simulink model "CAG_PH"  (R2020a)
settings: Solver=FixedStepAuto  StartTime=0.0  StopTime=10  FixedStep=1e-6  RelTol=1e-3  EnableMultiTasking=on
libraries: powerlib x23
settings Model: SimulationMode=accelerator  Creator=SINA  LastModifiedBy=ABO-CHIFA
settings DataIOCC: ReturnWorkspaceOutputs=off
settings OptimizationCC: LifeSpan=inf
settings DebuggingCC: SFUnexpectedBacktrackingDiag=warning  SFNoUnconditionalDefaultTransitionDiag=warning  ArithmeticOperatorsInVariantConditions=warning
settings SFSimCC: SimUseLocalCustomCode=off  CustomCodeUndefinedFunction=UseInterfaceOnly
settings RTWCC: RTWUseLocalCustomCode=off
settings CodeAppCC: StateflowObjectComments=on
settings GRTTargetCC: TargetLangStandard=C89/C90 (ANSI)
settings ConfigComp: CovMetricSettings=dw  CovHtmlReporting=on  CovSaveCumulativeToWorkspaceVar=on  CovSaveSingleToWorkspaceVar=on  CovExternalEMLEnable=off
settings SimscapeCC: SimscapeNormalizeSystem=off

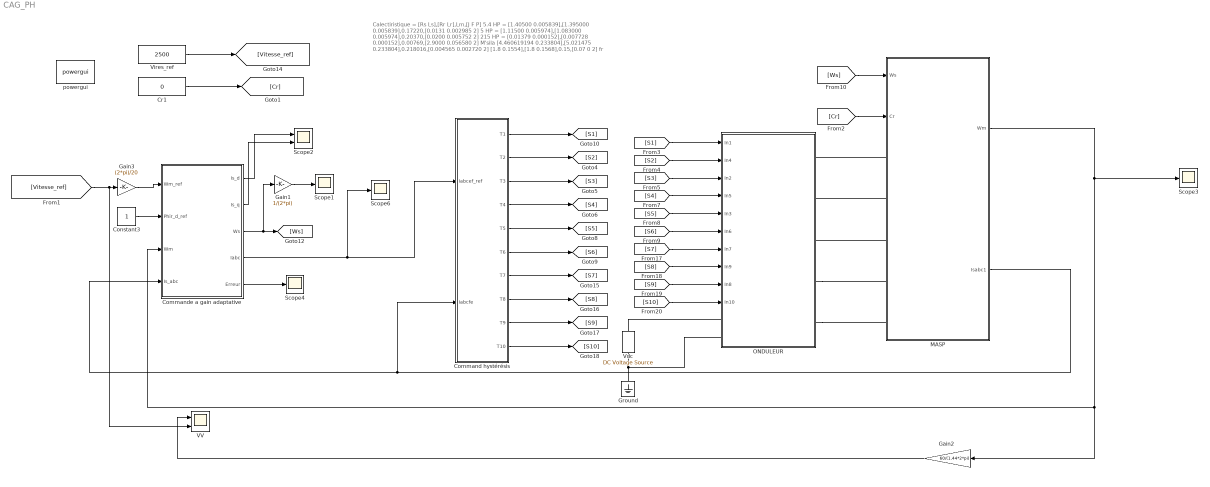
== system CAG_PH ==
  note: Calectiristique = [Rs Ls],[Rr Lr],Lm,[J F P]
      |
      | 5.4 HP = [1.40500 0.005839],[1.395000 0.005839],0.17220,[0.0131 0.002985 2]
      | 5 HP = [1.11500 0.005974],[1.083000 0.005974],0.20370,[0.0200 0.005752 2]
      | 215 HP = [0.01379 0.000152],[0.007728 0.000152],0.00769,[2.9000 0.056580 2]
      |
      | M'sila
      | [4.460619194 0.233804],[5.021475 0.233804],0.218016,[0.004565 0.002720 2]
      |
      | [1.8 0.1554],[1.8 0.1568],0.15,[0.07 0 2] fr
  Command hystérésis : Subsystem
  Commande a gain adaptative : Subsystem
  Constant3 : Constant
  Cr1 : Constant  Value=0
  Gain1 : Gain  Gain=1/(2*pi)
  Gain2 : Gain  Gain=60/(1.44*2*pi)
  Gain3 : Gain  Gain=(2*pi)/20
  Ground : powerlib/Elements/Ground  LConnTagsString=a
  MASP : Subsystem
  ONDULEUR : Subsystem
  Scope{1,3..4,6} (4 alike) : Scope
  Scope2 : Scope  NumInputPorts=2
  VV : Scope  NumInputPorts=2
  Vdc : powerlib/Electrical Sources/DC Voltage Source  Amplitude=650  Measurements=Voltage
  Vires_ref : Constant  Value=2500
  powergui : powerlib/powergui  Priority=1  SimulationMode=Discrete  SampleTime=1e-6  frequency=60  Iterations=50  frequencyindice=0  Pbase=100e6  ErrMax=1e-4  UnitsV=kV  UnitsW=MW  buscounter=0  FunctionMessages=off  echomessages=off  EnableUseOfTLC=off  CurrentSourceSwitches=off  DisableSnubberDevices=off  DisableRonSwitches=off  DisableVfSwitches=off  DisplayEquations=off  AutomaticDiscreteSolvers=off  SolverType=Tustin/Backward Euler (TBE)  Interpol=off  ExternalGateDelay=off  methode=off  Ts=0  x0status=blocks  SPID=off  SwTol=0  HookPort=off  NonlinearTolerance=1e-4  nMaxIteration=100  ContinueOnMaxIteration=off  RestoreLinks=warning  ResistiveCurrentMeasurement=off  Frange=[0:2:500]  Ylog=off  Xlog=on  ShowGrid=off  save=off  variable=ZData  structure=0  ZoomFFT=on  StartTime=0.0  cycles=1  DisplayStyle=1  fundamental=60  FreqAxis=off  MaxFrequency=1000  frequencyindicesteady=1  RmsSteady=1  display=off
  wires:
  Constant3/1 -> Commande a gain adaptative/2(Phir_d_ref)
  Commande a gain adaptative/3(Ws) -> [Ws], Gain1/1
  Commande a gain adaptative/4(Iabc) -> Command hystérésis/1(Iabcef_ref), Scope6/1
  Gain1/1 -> Scope1/1
  Commande a gain adaptative/1(Is_d) -> Scope2/1
  Commande a gain adaptative/2(Is_q) -> Scope2/2
  Commande a gain adaptative/5(Erreur) -> Scope4/1
  Cr1/1 -> [Cr]
  [Ws] -> MASP/1(Ws)
  [Cr] -> MASP/2(Cr)
  [Vitesse_ref] -> VV/2, Gain3/1
  Gain3/1 -> Commande a gain adaptative/1(Wm_ref)
  Gain2/1 -> VV/1
  MASP/1(Wm) -> Scope3/1, Gain2/1, Commande a gain adaptative/3(Wm)
  Vires_ref/1 -> [Vitesse_ref]
  [S1] -> ONDULEUR/1(In1)
  [S2] -> ONDULEUR/2(In4)
  [S10] -> ONDULEUR/10(In10)
  [S9] -> ONDULEUR/9(In8)
  [S3] -> ONDULEUR/3(In2)
  [S7] -> ONDULEUR/7(In7)
  [S6] -> ONDULEUR/6(In6)
  [S8] -> ONDULEUR/8(In9)
  [S4] -> ONDULEUR/4(In5)
  [S5] -> ONDULEUR/5(In3)
  Command hystérésis/2(T2) -> [S2]
  Command hystérésis/8(T8) -> [S8]
  Command hystérésis/9(T9) -> [S9]
  MASP/2(Isabc1) -> Command hystérésis/2(Iabcfe), Commande a gain adaptative/4(Is_abc)
  Command hystérésis/10(T10) -> [S10]
  Command hystérésis/1(T1) -> [S1]
  Command hystérésis/3(T3) -> [S3]
  Command hystérésis/5(T5) -> [S5]
  Command hystérésis/4(T4) -> [S4]
  Command hystérésis/7(T7) -> [S7]
  Command hystérésis/6(T6) -> [S6]
  connections:
  ONDULEUR/LConn2 -- Vdc/LConn1 -- Ground/LConn1
  Vdc/RConn1 -- ONDULEUR/LConn1
  MASP/LConn1 -- ONDULEUR/RConn1
  MASP/LConn2 -- ONDULEUR/RConn2
  MASP/LConn3 -- ONDULEUR/RConn3
  ONDULEUR/RConn4 -- MASP/LConn4
  ONDULEUR/RConn5 -- MASP/LConn5

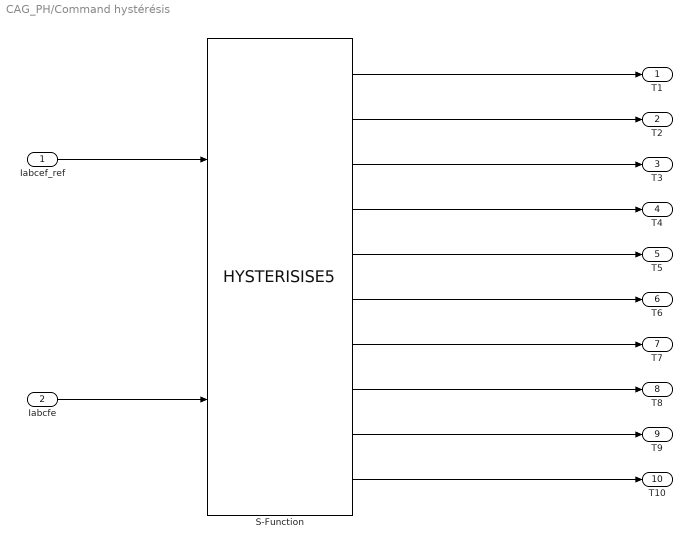
== system CAG_PH/Command hystérésis ==
  Iabcef_ref : Inport
  Iabcfe : Inport  Port=2
  S-Function : S-Function  FunctionName=HYSTERISISE5  Parameters=""  SFunctionDeploymentMode=off  EnableBusSupport=off
  T1 : Outport
  T2 : Outport  Port=2
  T3 : Outport  Port=3
  T4 : Outport  Port=4
  T5 : Outport  Port=5
  T6 : Outport  Port=6
  T7 : Outport  Port=7
  T8 : Outport  Port=8
  T9 : Outport  Port=9
  T10 : Outport  Port=10
  wires:
  Iabcef_ref/1 -> S-Function/1
  Iabcfe/1 -> S-Function/2
  S-Function/1 -> T1/1
  S-Function/2 -> T2/1
  S-Function/3 -> T3/1
  S-Function/4 -> T4/1
  S-Function/5 -> T5/1
  S-Function/6 -> T6/1
  S-Function/7 -> T7/1
  S-Function/8 -> T8/1
  S-Function/9 -> T9/1
  S-Function/10 -> T10/1

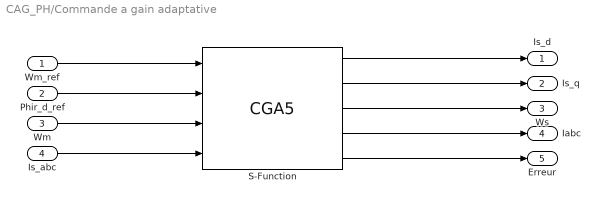
== system CAG_PH/Commande a gain adaptative ==
  Wm_ref : Inport
  Phir_d_ref : Inport  Port=2
  Wm : Inport  Port=3
  Is_abc : Inport  Port=4
  S-Function : S-Function  FunctionName=CGA5  Parameters=[1.40500 0.005839],[1.395000 0.005839],0.17220,[0.0131 0.002985 2]  SFunctionDeploymentMode=off  EnableBusSupport=off
  Is_d : Outport
  Is_q : Outport  Port=2
  Ws : Outport  Port=3
  Iabc : Outport  Port=4
  Erreur : Outport  Port=5
  wires:
  S-Function/4 -> Iabc/1
  S-Function/3 -> Ws/1
  S-Function/2 -> Is_q/1
  S-Function/1 -> Is_d/1
  Wm/1 -> S-Function/3
  Phir_d_ref/1 -> S-Function/2
  Wm_ref/1 -> S-Function/1
  S-Function/5 -> Erreur/1
  Is_abc/1 -> S-Function/4

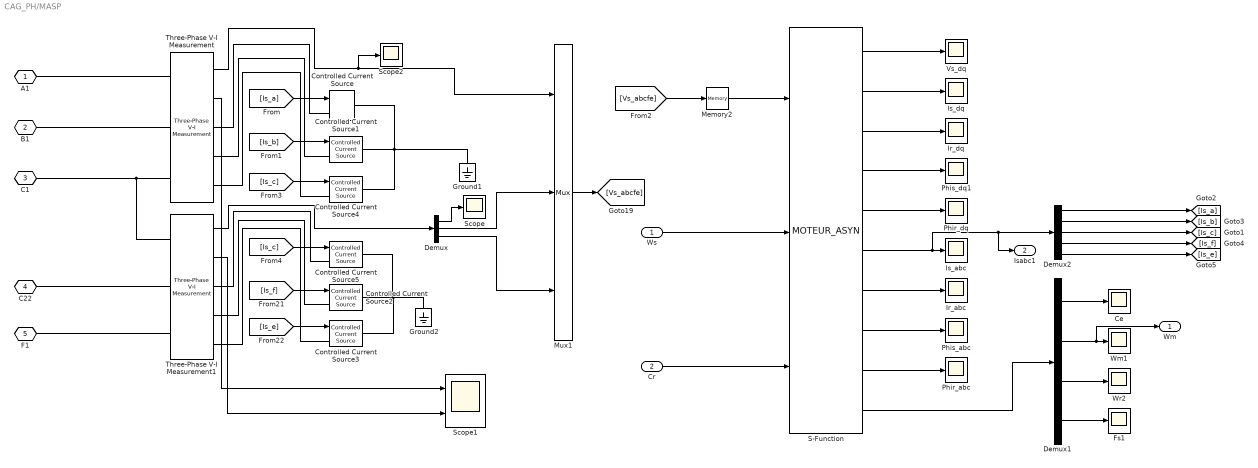
== system CAG_PH/MASP ==
  Ws : Inport
  Cr : Inport  Port=2
  Ce : Scope
  Controlled Current Source{,1..5} (6 alike) : powerlib/Electrical Sources/Controlled Current Source  Initialize=off  Source_Type=AC  Amplitude=0  Phase=0  Frequency=50  Measurements=None
  Demux : Demux  Outputs=3
  Demux1 : Demux
  Demux2 : Demux  Outputs=5
  Fs1 : Scope
  Ground1 : powerlib/Elements/Ground  LConnTagsString=a
  Ground2 : powerlib/Elements/Ground  LConnTagsString=a
  Ir_abc : Scope
  Ir_dq : Scope
  Is_abc : Scope
  Is_dq : Scope
  Memory2 : Memory
  Mux1 : Mux  Inputs=3
  Phir_abc : Scope
  Phir_dq : Scope
  Phis_abc : Scope
  Phis_dq1 : Scope
  S-Function : S-Function  FunctionName=MOTEUR_ASYN  Parameters=[1.40500 0.005839],[1.395000 0.005839],0.17220,[0.0131 0.002985 2]  SFunctionDeploymentMode=off  EnableBusSupport=off
  Scope : Scope
  Scope1 : Scope  NumInputPorts=2
  Scope2 : Scope
  Three-Phase V-I Measurement : powerlib/Measurements/Three-Phase V-I Measurement  VoltageMeasurement=phase-to-ground  SetLabelV=off  LabelV=Vabc  Vpu=off  VpuLL=off  CurrentMeasurement=yes  SetLabelI=off  LabelI=Iabc  Ipu=off  Pbase=100e6  Vbase=500e3  OutputType=Complex  PhasorSimulation=off  PSBequivalent=0
  Three-Phase V-I Measurement1 : powerlib/Measurements/Three-Phase V-I Measurement  VoltageMeasurement=phase-to-ground  SetLabelV=off  LabelV=Vabc  Vpu=off  VpuLL=off  CurrentMeasurement=yes  SetLabelI=off  LabelI=Iabc  Ipu=off  Pbase=100e6  Vbase=500e3  OutputType=Complex  PhasorSimulation=off  PSBequivalent=0
  Vs_dq : Scope
  Wm1 : Scope
  Wr2 : Scope
  A1 : PMIOPort  Tag=PMCPort  Side=Left
  B1 : PMIOPort  Tag=PMCPort  Port=2  Side=Left
  C1 : PMIOPort  Tag=PMCPort  Port=3  Side=Left
  C22 : PMIOPort  Tag=PMCPort  Port=4  Side=Left
  F1 : PMIOPort  Tag=PMCPort  Port=5  Side=Left
  Wm : Outport
  Isabc1 : Outport  Port=2
  wires:
  Demux1/2 -> Wm/1, Wm1/1
  Demux1/3 -> Wr2/1
  Ws/1 -> S-Function/2
  S-Function/7 -> Ir_abc/1
  S-Function/9 -> Phir_abc/1
  S-Function/2 -> Is_dq/1
  Demux1/4 -> Fs1/1
  S-Function/6 -> Isabc1/1, Demux2/1, Is_abc/1
  Demux1/1 -> Ce/1
  S-Function/5 -> Phir_dq/1
  S-Function/10 -> Demux1/1
  S-Function/8 -> Phis_abc/1
  S-Function/4 -> Phis_dq1/1
  S-Function/1 -> Vs_dq/1
  Cr/1 -> S-Function/3
  S-Function/3 -> Ir_dq/1
  Demux2/1 -> [Is_a]
  [Vs_abcfe] -> Memory2/1
  Memory2/1 -> S-Function/1
  [Is_e] -> Controlled Current Source3/1
  [Is_b] -> Controlled Current Source1/1
  [Is_f] -> Controlled Current Source2/1
  Three-Phase V-I Measurement1/1 -> Demux/1
  Three-Phase V-I Measurement/1 -> Scope2/1, Mux1/1
  [Is_a] -> Controlled Current Source/1
  Mux1/1 -> [Vs_abcfe]
  Demux2/5 -> [Is_e]
  Demux2/4 -> [Is_f]
  Demux2/3 -> [Is_c]
  Demux2/2 -> [Is_b]
  [Is_c] -> Controlled Current Source4/1
  [Is_c] -> Controlled Current Source5/1
  Demux/2 -> Mux1/2
  Demux/3 -> Mux1/3
  Demux/1 -> Scope/1
  Three-Phase V-I Measurement/2 -> Scope1/1
  Three-Phase V-I Measurement1/2 -> Scope1/2
  connections:
  Controlled Current Source1/RConn1 -- Ground1/LConn1 -- Controlled Current Source/RConn1 -- Controlled Current Source4/RConn1
  C1/RConn1 -- Three-Phase V-I Measurement1/LConn1 -- Three-Phase V-I Measurement/LConn3
  Controlled Current Source3/RConn1 -- Controlled Current Source2/RConn1 -- Controlled Current Source5/RConn1 -- Ground2/LConn1
  B1/RConn1 -- Three-Phase V-I Measurement/LConn2
  A1/RConn1 -- Three-Phase V-I Measurement/LConn1
  Three-Phase V-I Measurement/RConn2 -- Controlled Current Source1/LConn1
  Three-Phase V-I Measurement/RConn1 -- Controlled Current Source/LConn1
  Controlled Current Source4/LConn1 -- Three-Phase V-I Measurement/RConn3
  Controlled Current Source3/LConn1 -- Three-Phase V-I Measurement1/RConn3
  Controlled Current Source2/LConn1 -- Three-Phase V-I Measurement1/RConn2
  F1/RConn1 -- Three-Phase V-I Measurement1/LConn3
  C22/RConn1 -- Three-Phase V-I Measurement1/LConn2
  Controlled Current Source5/LConn1 -- Three-Phase V-I Measurement1/RConn1

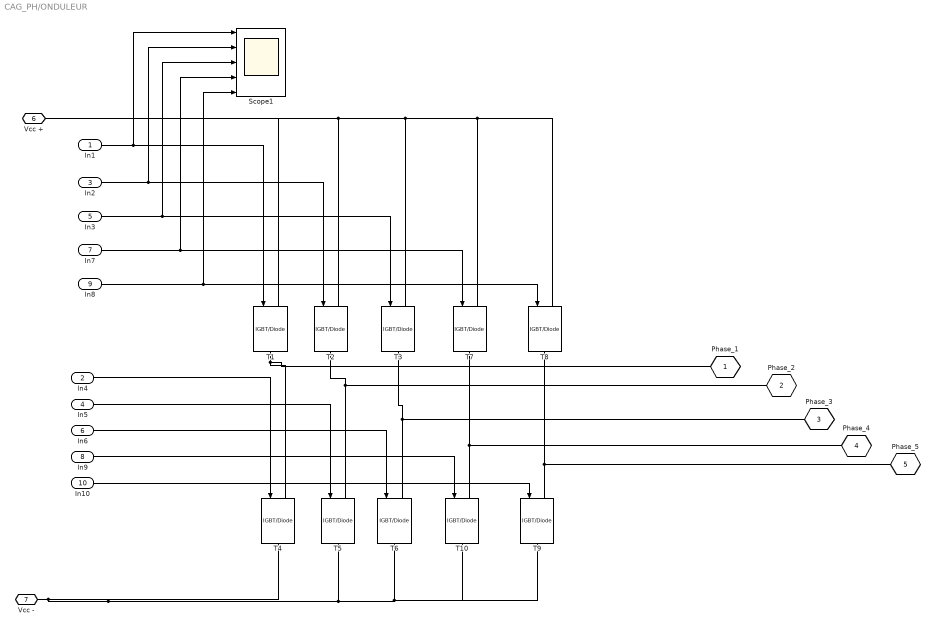
== system CAG_PH/ONDULEUR ==
  In1 : Inport
  In4 : Inport  Port=2
  In2 : Inport  Port=3
  In5 : Inport  Port=4
  In3 : Inport  Port=5
  In6 : Inport  Port=6
  In7 : Inport  Port=7
  In9 : Inport  Port=8
  In8 : Inport  Port=9
  In10 : Inport  Port=10
  Scope1 : Scope  NumInputPorts=5
  T{1..10} (10 alike) : powerlib/Power Electronics/IGBT//Diode  Ron=1e-3  Rs=1e5  Cs=inf  Measurements=off
  Phase_1 : PMIOPort  Tag=PMCPort  Side=Right
  Phase_2 : PMIOPort  Tag=PMCPort  Port=2  Side=Right
  Phase_3 : PMIOPort  Tag=PMCPort  Port=3  Side=Right
  Phase_4 : PMIOPort  Tag=PMCPort  Port=4  Side=Right
  Phase_5 : PMIOPort  Tag=PMCPort  Port=5  Side=Right
  Vcc + : PMIOPort  Port=6  Side=Left
  Vcc - : PMIOPort  Port=7  Side=Left
  wires:
  In1/1 -> Scope1/1, T1/1
  In9/1 -> T10/1
  In5/1 -> T5/1
  In4/1 -> T4/1
  In3/1 -> Scope1/3, T3/1
  In8/1 -> Scope1/5, T8/1
  In7/1 -> Scope1/4, T7/1
  In10/1 -> T9/1
  In6/1 -> T6/1
  In2/1 -> Scope1/2, T2/1
  connections:
  T6/LConn1 -- T3/RConn1 -- Phase_3/RConn1
  T5/LConn1 -- T2/RConn1 -- Phase_2/RConn1
  Phase_4/RConn1 -- T10/LConn1 -- T7/RConn1
  Vcc -/RConn1 -- T10/RConn1 -- T9/RConn1 -- T6/RConn1 -- T5/RConn1 -- T4/RConn1
  T7/LConn1 -- T8/LConn1 -- T3/LConn1 -- Vcc +/RConn1 -- T1/LConn1 -- T2/LConn1
  T9/LConn1 -- Phase_5/RConn1 -- T8/RConn1
  T1/RConn1 -- T4/LConn1 -- Phase_1/RConn1
